simulink model "mqtt_simulink_24b"  (R2024b)
settings: Solver=ode5  StartTime=0.0  StopTime=inf  RelTol=1e-3
PreLoadFcn:
  | modellSti = fileparts(which(bdroot));
  | addpath(genpath(fullfile(modellSti, 'mqtt')));
  | addpath(genpath('mqtt'));
PostLoadFcn:
  | modellSti = fileparts(which(bdroot));
  | addpath(genpath(fullfile(modellSti, 'mqtt')));
  | addpath(genpath('mqtt'));
InitFcn:
  | modellSti = fileparts(which(bdroot));
  | addpath(genpath(fullfile(modellSti, 'mqtt')));
  | addpath(genpath('mqtt'));
libraries: slpidlib x1, read x1, init x1, send x1
settings Model: Creator=adriaeik  LastModifiedBy=eikel
settings HardwareCC: ProdBitPerLong=64  ProdHWDeviceType=Intel->x86-64 (Linux 64)
settings RTWCC: Description=Simulink Desktop Real-Time  SystemTargetFile=sldrt.tlc  TemplateMakefile=sldrt.tmf  TargetLang=C++  RTWCompilerOptimization=on
settings CodeAppCC: MaxIdLength=95
settings SimulinkDesktopRealTimeCC: TargetLibSuffix=_sldrt.a  TargetPreCompLibLocation=C:\Program Files\MATLAB\R2024a\toolbox\sldrt\lib\win64  TargetLangStandard=C++11 (ISO)  CCListing=on  RebuildAll=on

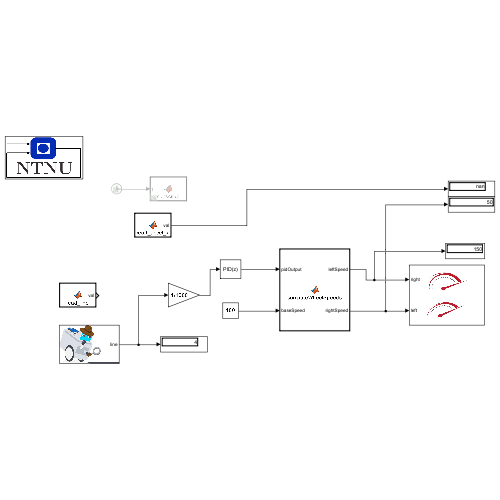
[thumbnail: Simulink's stored preview of the top-level diagram]
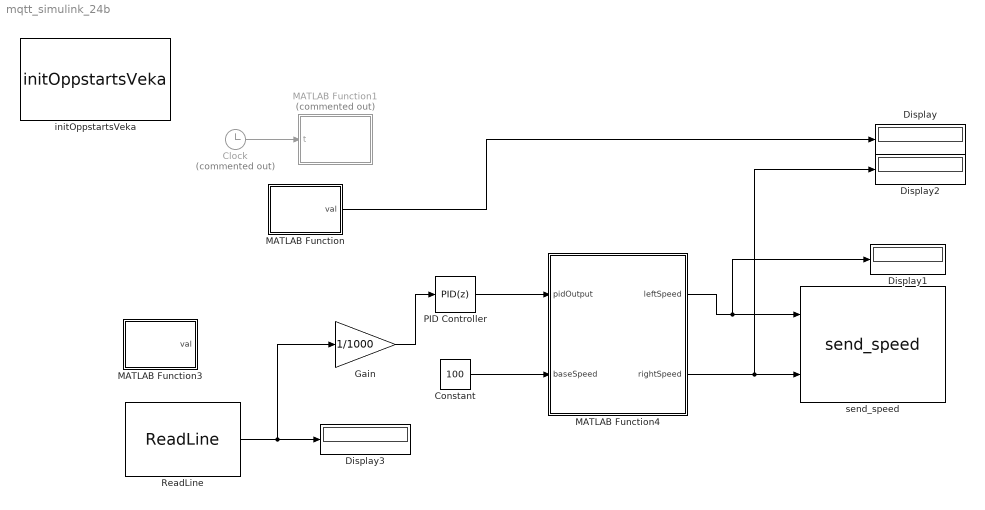
== system mqtt_simulink_24b ==
  Clock : Clock  Commented=on
  Constant : Constant  Value=100
  Display{,1..3} (4 alike) : Display
      Display2 settings: Format=decimal (Stored Integer)
  Gain : Gain  Gain=1/1000
  MATLAB Function : MATLAB Function  TreatAsAtomicUnit=on
  MATLAB Function1 : MATLAB Function  Commented=on  TreatAsAtomicUnit=on
  MATLAB Function3 : MATLAB Function  TreatAsAtomicUnit=on
  MATLAB Function4 : MATLAB Function  TreatAsAtomicUnit=on
  PID Controller : slpidlib/PID Controller  Controller=PID  Form=Parallel  TimeDomain=Discrete-time  UseExternalTs=off  SampleTime=0.12  IntegratorMethod=Forward Euler  FilterMethod=Forward Euler  ControllerParametersSource=internal  P=30  I=10  UseKiTs=off  D=0  UseExternalDerivativeSource=off  N=100  UseFilter=on  TunerSelectOption=Transfer Function Based (PID Tuner App)  InitialConditionSource=internal  InitialConditionForIntegrator=0  InitialConditionForFilter=0  DifferentiatorICPrevScaledInput=0  ExternalReset=none  TrackingMode=off  Kt=1  LimitOutput=off  SatLimitsSource=internal  UpperSaturationLimit=inf  LowerSaturationLimit=-inf  LinearizeAsGain=on  AntiWindupMode=none  Kb=1  LimitIntegrator=off  UpperIntegratorSaturationLimit=inf  LowerIntegratorSaturationLimit=-inf  POutMin=[]  POutMax=[]  IOutMin=[]  IOutMax=[]  DOutMin=[]  DOutMax=[]  NOutMin=[]  NOutMax=[]  SumOutMin=[]  SumOutMax=[]  SaturationOutMin=[]  SaturationOutMax=[]  PParamMin=[]  PParamMax=[]  IParamMin=[]  IParamMax=[]  DParamMin=[]  DParamMax=[]  NParamMin=[]  NParamMax=[]  KbParamMin=[]  KbParamMax=[]  KtParamMin=[]  KtParamMax=[]  KbOutMin=[]  KbOutMax=[]  KtOutMin=[]  KtOutMax=[]  IntegratorOutMin=[]  IntegratorOutMax=[]  FilterOutMin=[]  FilterOutMax=[]  SumI1OutMin=[]  SumI1OutMax=[]  SumI2OutMin=[]  SumI2OutMax=[]  SumI3OutMin=[]  SumI3OutMax=[]  SumI4OutMin=[]  SumI4OutMax=[]  SumDOutMin=[]  SumDOutMax=[]  DifferentiatorOutMin=[]  DifferentiatorOutMax=[]  FilterDiffOutCoefMin=[]  FilterDiffOutCoefMax=[]  ReciprocalOutMin=[]  ReciprocalOutMax=[]  SumDenOutMin=[]  SumDenOutMax=[]  SumNumOutMin=[]  SumNumOutMax=[]  DivideOutMin=[]  DivideOutMax=[]  UdiffTsProdOutMin=[]  UdiffTsProdOutMax=[]  NTsProdOutMin=[]  NTsProdOutMax=[]  UintegralTsProdOutMin=[]  UintegralTsProdOutMax=[]  UngainTsProdOutMin=[]  UngainTsProdOutMax=[]  ClampingZeroOutDataTypeStr=Inherit: Inherit via back propagation  ClampingZeroOutMin=[]  ClampingZeroOutMax=[]  FilterDenConstantOutDataTypeStr=Inherit: Inherit via back propagation  FilterDenConstantOutMin=[]  FilterDenConstantOutMax=[]  PCopyOutDataTypeStr=Inherit: Inherit via back propagation  PCopyOutMin=[]  PCopyOutMax=[]  NCopyOutDataTypeStr=Inherit: Inherit via back propagation  NCopyOutMin=[]  NCopyOutMax=[]  IntegratorContinuousStateAttributes=''  IntegratorStateMustResolveToSignalObject=off  IntegratorRTWStateStorageClass=Auto  FilterContinuousStateAttributes=''  FilterStateMustResolveToSignalObject=off  FilterRTWStateStorageClass=Auto  ParallelPVariant=InternalParameters  IdealPVariant=Disabled  IVariant=InternalParameters  DVariant=InternalParameters  IntegratorVariant=Discrete  SatVariant=Disabled  AWVariant=Passthrough  PCopyVariant=Disabled  TRVariant=Disabled  FdbkBlocksVariant=Forward  IdealPFdbkVariant=Disabled  SatFdbkVariant=Disabled  DerivativeFilterVariant=ForwardEulerFilter  NVariant=InternalParameters  NCopyVariant=Disabled  FilterICVariant=InternalICsFilter  IntegratorICVariant=InternalICs  ExternalResetVariant=Disabled  TRSumVariant=Passthrough  SumFdbkVariant=Disabled  SumVariant=Sum_PID  TsampFilterVariant=InternalTs  TsampNgainVariant=Passthrough  TsampIntegralVariant=Disabled_SignalSpec  ExternalSaturationOutDataTypeStr=Inherit: Same as second input  DerivativeSourceVariant=ErrorSignal  PreIntVariant=InternalPreInt
  ReadLine : read/ReadLine
  initOppstartsVeka : init/initOppstartsVeka  carID=14
  send_speed : send/send_speed  SystemSampleTime=-1  VariantActivationTime=update diagram  AllowFlexibleInterface=on  Latency=0  AutoFrameSizeCalculation=off
  wires:
  MATLAB Function/1(val) -> Display/1
  Clock/1 -> MATLAB Function1/1(t)
  MATLAB Function4/1(leftSpeed) -> Display1/1, send_speed/1
  MATLAB Function4/2(rightSpeed) -> Display2/1, send_speed/2
  PID Controller/1 -> MATLAB Function4/1(pidOutput)
  Constant/1 -> MATLAB Function4/2(baseSpeed)
  Gain/1 -> PID Controller/1
  ReadLine/1 -> Gain/1, Display3/1

== matlab function mqtt_simulink_24b/MATLAB Function ==
  data: val output
function val = read_accel_x()
    coder.extrinsic('get_accel_x');  % merk: dette peikar på .m-fila di
    val = 0;                         % initier output
    val = get_accel_x();            % kall den eksterne funksjonen
end

== matlab function mqtt_simulink_24b/MATLAB Function3 ==
  data: val output
function val = read_line()
    coder.extrinsic('get_line');  % merk: dette peikar på .m-fila di
    val =0;                         % initier output
    val = get_line();            % kall den eksterne funksjonen
end

== matlab function mqtt_simulink_24b/MATLAB Function4 ==
  data: pidOutput input; leftSpeed output; baseSpeed input; rightSpeed output
function [leftSpeed, rightSpeed] = computeWheelSpeeds(pidOutput, baseSpeed)
% Funksjon for å konvertere PID-utslag til motorhastigheiter
% 
% INN:
%   pidOutput:    Styresignal frå PID-regulator, positivt for høgre sving
%   baseSpeed:    Grunnhastigheit bilen skal ha når den er på linja
%
% UT:
%   leftSpeed:    Hastigheit venstre motor
%   rightSpeed:   Hastigheit høgre motor

    % Begrens maks differanse (unngå for høg sving)
    maxDiff = baseSpeed/2; % kan justerast etter behov

    % Klipp PID-utslag om nødvendig
    correction = max(-maxDiff, min(maxDiff, pidOutput));

    % Juster hastigheiter
    leftSpeed = baseSpeed + correction;
    rightSpeed = baseSpeed - correction;
end

== matlab function mqtt_simulink_24b/MATLAB Function1 ==
  data: t input
function subscribe(t)
    coder.extrinsic('mqtt_subscribe');  % merk: dette peikar på .m-fila di
   if mod(t,10)==0
       get_accel_x();            % kall den eksterne funksjonen
   end
end
